simulink model "gm_pwm"  (R2017a)
settings: Solver=FixedStepAuto  StartTime=0.0  StopTime=.00001  FixedStep=1/100e6  RelTol=1e-3  EnableMultiTasking=on
settings Model: Creator=dskaputa  LastModifiedBy=zdw7287
settings OptimizationCC: BlockReduction=off  ConditionallyExecuteInputs=off  LifeSpan=inf
settings DebuggingCC: InheritedTsInSrcMsg=none  SFUnexpectedBacktrackingDiag=warning  SFNoUnconditionalDefaultTransitionDiag=warning  SFExecutionAtInitializationDiag=none
settings GRTTargetCC: TargetLangStandard=C89/C90 (ANSI)
settings ConfigComp: CovMetricSettings=dw  CovHtmlReporting=on  CovSaveCumulativeToWorkspaceVar=on  CovSaveSingleToWorkspaceVar=on  CovExternalEMLEnable=off

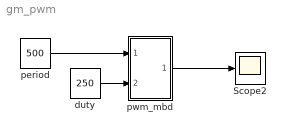
== system gm_pwm ==
  Scope2 : Scope
  "duty " : Constant  Value=250  OutDataTypeStr=fixdt(0,27,0)  SampleTime=-1
  period : Constant  Value=500  OutDataTypeStr=fixdt(0,27,0)  SampleTime=-1
  pwm_mbd : Subsystem
  wires:
  "duty "/1 -> pwm_mbd/2(duty)
  period/1 -> pwm_mbd/1(period)
  pwm_mbd/1(pwm_output) -> Scope2/1

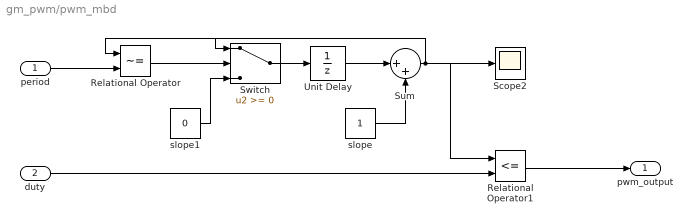
== system gm_pwm/pwm_mbd ==
  period : Inport  SampleTime=1e-08
  duty : Inport  Port=2  SampleTime=1e-08
  Relational Operator : RelationalOperator  Operator=~=  OutDataTypeStr=boolean  RndMeth=Nearest
  Relational Operator1 : RelationalOperator  Operator=<=  OutDataTypeStr=boolean  RndMeth=Nearest
  Scope2 : Scope
  Sum : Sum  Inputs=|++  AccumDataTypeStr=fixdt(0,27,0)  OutDataTypeStr=fixdt(0,27,0)  SaturateOnIntegerOverflow=on
  Switch : Switch
  Unit Delay : UnitDelay  SampleTime=-1
  slope : Constant  OutDataTypeStr=fixdt(0,10,0)  SampleTime=-1
  slope1 : Constant  Value=0  OutDataTypeStr=fixdt(0,10,0)  SampleTime=-1
  pwm_output : Outport
  wires:
  period/1 -> Relational Operator/2
  duty/1 -> Relational Operator1/2
  Relational Operator/1 -> Switch/2
  Relational Operator1/1 -> pwm_output/1
  Sum/1 -> Switch/1, Relational Operator1/1, Relational Operator/1, Scope2/1
  Switch/1 -> Unit Delay/1
  Unit Delay/1 -> Sum/1
  slope/1 -> Sum/2
  slope1/1 -> Switch/3
